simulink model "jakismodel"  (R2024b)
settings: Solver=VariableStepAuto  StartTime=0.0  StopTime=10.0  RelTol=1e-3
values from neighbouring files (symbols this model uses):
  kp = wartosci_wyznaczone(1)    [commandlineinterpretation2.m]    (also in flc_error_ffunc.m = x(1))
  ti = wartosci_wyznaczone(2)    [commandlineinterpretation2.m]    (also in flc_error_ffunc.m = x(2))
settings Model: Creator=maciejklossek  LastModifiedBy=maciejklossek

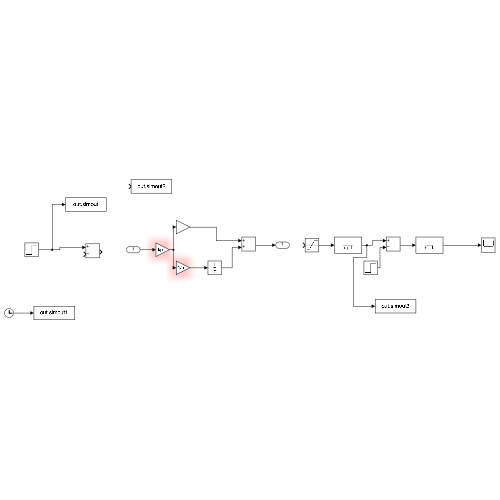
[thumbnail: Simulink's stored preview of the top-level diagram]
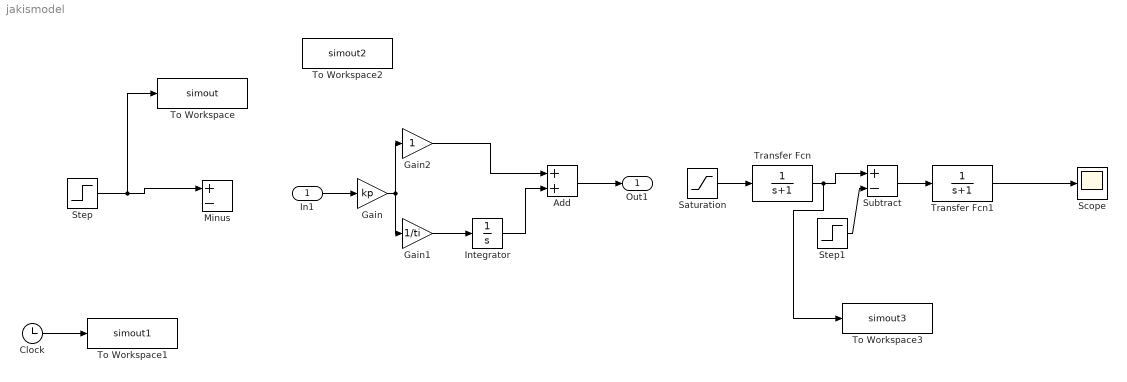
== system jakismodel ==
  In1 : Inport
  Add : Sum
  Clock : Clock
  Gain : Gain  Gain=kp
  Gain1 : Gain  Gain=1/ti
  Gain2 : Gain
  Integrator : Integrator
  Minus : Sum  Inputs=+-
  Saturation : Saturate
  Scope : Scope
  Step : Step  Time=0.1  After=0.25  SampleTime=0
  Step1 : Step  SampleTime=0
  Subtract : Sum  Inputs=+-
  To Workspace : ToWorkspace  VariableName=simout  SaveFormat=Timeseries  SampleTime=-1
  To Workspace1 : ToWorkspace  VariableName=simout1  SaveFormat=Timeseries  SampleTime=-1
  To Workspace2 : ToWorkspace  VariableName=simout2  SaveFormat=Timeseries  SampleTime=-1
  To Workspace3 : ToWorkspace  VariableName=simout3  SaveFormat=Timeseries  SampleTime=-1
  Transfer Fcn : TransferFcn  Denominator=[1 1]
  Transfer Fcn1 : TransferFcn  Denominator=[1 1]
  Out1 : Outport
  wires:
  Step/1 -> Minus/1, To Workspace/1
  Clock/1 -> To Workspace1/1
  In1/1 -> Gain/1
  Gain/1 -> Gain2/1, Gain1/1
  Gain1/1 -> Integrator/1
  Add/1 -> Out1/1
  Integrator/1 -> Add/2
  Gain2/1 -> Add/1
  Saturation/1 -> Transfer Fcn/1
  Transfer Fcn/1 -> To Workspace3/1, Subtract/1
  Step1/1 -> Subtract/2
  Subtract/1 -> Transfer Fcn1/1
  Transfer Fcn1/1 -> Scope/1
